simulink model "Impedance_control_RR"  (R2016b)
settings: Solver=VariableStepAuto  StartTime=0.0  StopTime=1.0  RelTol=1e-3
settings Model: Creator=Roozbeh  LastModifiedBy=Roozbeh

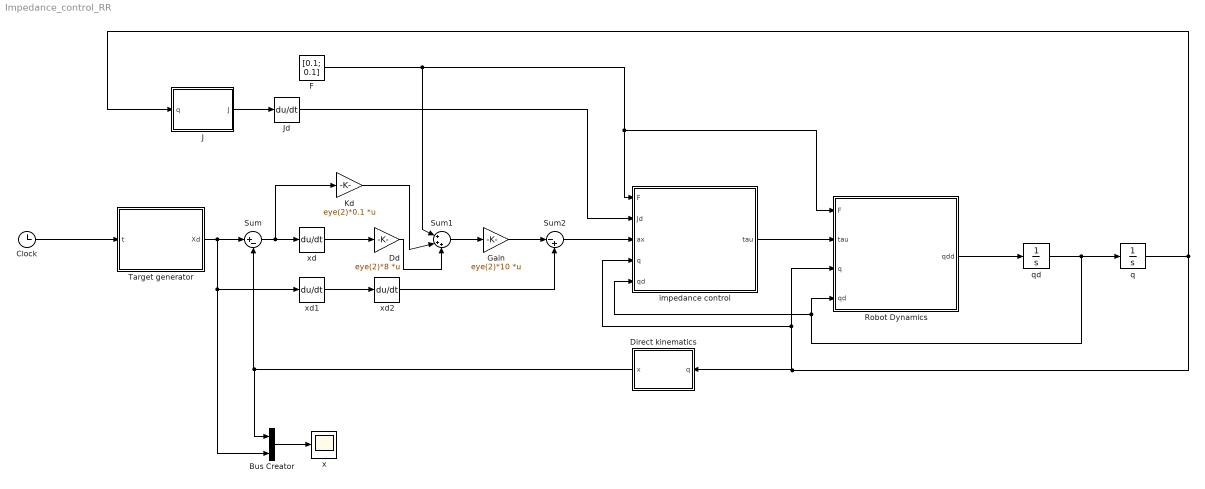
== system Impedance_control_RR ==
  Bus Creator : BusCreator  Inputs=2
  Clock : Clock
  Dd : Gain  Gain=eye(2)*8  Multiplication=Matrix(K*u)
  Direct kinematics : MATLAB Function  TreatAsAtomicUnit=on
  F : Constant  Value=[0.1; 0.1]
  Gain : Gain  Gain=eye(2)*10  Multiplication=Matrix(K*u)
  J : MATLAB Function  TreatAsAtomicUnit=on
  Jd : Derivative
  Kd : Gain  Gain=eye(2)*0.1  Multiplication=Matrix(K*u)
  Robot Dynamics : MATLAB Function  TreatAsAtomicUnit=on
  Sum : Sum  Inputs=|+-
  Sum1 : Sum  Inputs=|+++
  Sum2 : Sum  Inputs=|-+
  Target generator : MATLAB Function  TreatAsAtomicUnit=on
  impedance control : MATLAB Function  TreatAsAtomicUnit=on
  q : Integrator  InitialCondition=[pi/3; -2*pi/3]*1
  qd : Integrator  InitialCondition=[0; 0]
  x : Scope
  xd : Derivative
  xd1 : Derivative
  xd2 : Derivative
  wires:
  Clock/1 -> Target generator/1(t)
  Robot Dynamics/1(qdd) -> qd/1
  qd/1 -> q/1, impedance control/5(qd), Robot Dynamics/4(qd)
  q/1 -> Direct kinematics/1(q), impedance control/4(q), Robot Dynamics/3(q), J/1(q)
  Target generator/1(Xd) -> xd1/1, Bus Creator/2, Sum/1
  Direct kinematics/1(x) -> Bus Creator/1, Sum/2
  Sum/1 -> Kd/1, xd/1
  xd/1 -> Dd/1
  impedance control/1(tau) -> Robot Dynamics/2(tau)
  F/1 -> Sum1/1, Robot Dynamics/1(F), impedance control/1(F)
  Sum1/1 -> Gain/1
  J/1(J) -> Jd/1
  Jd/1 -> impedance control/2(Jd)
  Bus Creator/1 -> x/1
  xd1/1 -> xd2/1
  Dd/1 -> Sum1/3
  Kd/1 -> Sum1/2
  Gain/1 -> Sum2/1
  Sum2/1 -> impedance control/3(ax)
  xd2/1 -> Sum2/2

== matlab function Impedance_control_RR/impedance control ==
  data: F input; Jd input; ax input; q input; qd input; tau output
function tau = fcn(F, Jd, ax, q, qd)

Md = eye(2)*0.1;
L1 = 0.2;
L2 = 0.2;

Lc1 = L1/2;
Lc2 = L2/2;

g = 9.81;
m1 = 1;
m2 = 1;
I1 = 0.003;
I2 = 0.003;

q1 = q(1);
q2 = q(2);
qd1 = qd(1);
qd2 = qd(2);

Jc1 = [-Lc1*sin(q1) 0; Lc1*cos(q1) 0];
Jc2 = [-L1*sin(q1) - Lc2*sin(q1+q2), -Lc2*sin(q1+q2); ...
        L1*cos(q1) + Lc2*cos(q1+q2), Lc2*cos(q1+q2)];

M = m1*(Jc1')*Jc1 + m2*(Jc2')*Jc2 + [I1+I2 I2; I2 I2];

h = -m2*L1*Lc2*sin(q2);
C = [h*qd2 h*qd2+h*qd1; -h*qd1 0];

G = [(m1*Lc1 + m2*L1)*g*cos(q1) + m2*Lc2*g*cos(q1+q2); m2*Lc2*g*cos(q1+q2)];

J = [-L1*sin(q1) - L2*sin(q1+q2), -L2*sin(q1+q2); ...
        L1*cos(q1) + L2*cos(q1+q2), L2*cos(q1+q2)];

hN = C*qd + G;

tau = hN - M*pinv(J)*Jd*qd - M*pinv(J)*pinv(Md)*ax + (M*pinv(J)*pinv(Md)-transpose(J))*F;

== matlab function Impedance_control_RR/Target generator ==
  data: t input; Xd output
function Xd = fcn(t)

Xd = [0.2 + 0.1*(6*t^5 - 15*t^4 + 10*t^3); 0];
% Xd = [0.4; 0];


% L1 = 0.2;
% L2 = 0.2;
% q1 = 0.2 + 0.1*(6*t^5 - 15*t^4 + 10*t^3);
% q2 = 0;
% Xd = [L1*cos(q1) + L2*cos(q1+q2); L1*sin(q1) + L2*sin(q1+q2)];

== matlab function Impedance_control_RR/Robot Dynamics ==
  data: F input; tau input; q input; qd input; qdd output
function qdd = fcn(F, tau, q, qd)

L1 = 0.2;
L2 = 0.2;

Lc1 = L1/2;
Lc2 = L2/2;

g = 9.81;
m1 = 1;
m2 = 1;
I1 = 0.003;
I2 = 0.003;

q1 = q(1);
q2 = q(2);
qd1 = qd(1);
qd2 = qd(2);

Jc1 = [-Lc1*sin(q1) 0; Lc1*cos(q1) 0];
Jc2 = [-L1*sin(q1) - Lc2*sin(q1+q2), -Lc2*sin(q1+q2); ...
        L1*cos(q1) + Lc2*cos(q1+q2), Lc2*cos(q1+q2)];

D = m1*(Jc1')*Jc1 + m2*(Jc2')*Jc2 + [I1+I2 I2; I2 I2];

h = -m2*L1*Lc2*sin(q2);
C = [h*qd2 h*qd2+h*qd1; -h*qd1 0];

G_mat = [(m1*Lc1 + m2*L1)*g*cos(q1) + m2*Lc2*g*cos(q1+q2); m2*Lc2*g*cos(q1+q2)];

J = [-L1*sin(q1) - L2*sin(q1+q2), -L2*sin(q1+q2); ...
        L1*cos(q1) + L2*cos(q1+q2), L2*cos(q1+q2)];


qdd = pinv(D)*(tau + transpose(J)*F - C*qd - G_mat);

== matlab function Impedance_control_RR/Direct kinematics ==
  data: q input; x output
function x = fcn(q)
L1 = 0.2;
L2 = 0.2;
q1 = q(1);
q2 = q(2);
x = [L1*cos(q1) + L2*cos(q1+q2); L1*sin(q1) + L2*sin(q1+q2)];

== matlab function Impedance_control_RR/J ==
  data: q input; J output
function J = fcn(q)
L1 = 0.2;
L2 = 0.2;
q1 = q(1);
q2 = q(2);
J = [-L1*sin(q1) - L2*sin(q1+q2), -L2*sin(q1+q2); ...
        L1*cos(q1) + L2*cos(q1+q2), L2*cos(q1+q2)];
